simulink model "model6krata"  (Simulink 6.6)
settings: Solver=ode45  StartTime=0.0  StopTime=700  MaxStep=0.01  MinStep=0.001  RelTol=1e-6
values from neighbouring files (symbols this model uses):
  c1 = 8    [dane6krata.m]
  c2 = 5    [dane6krata.m]
  mi1 = 1    [dane6krata.m]
  mi2 = 2    [dane6krata.m]
  q = 1    [dane6krata.m]
undefined symbols (not defined in the file or in its folder): sgn
settings Model: Creator=Administrator  LastModifiedBy=Damian
settings DataIOCC: LimitDataPoints=off
settings GRTTargetCC: TargetFcnLib=ansi_tfl_table_tmw.mat

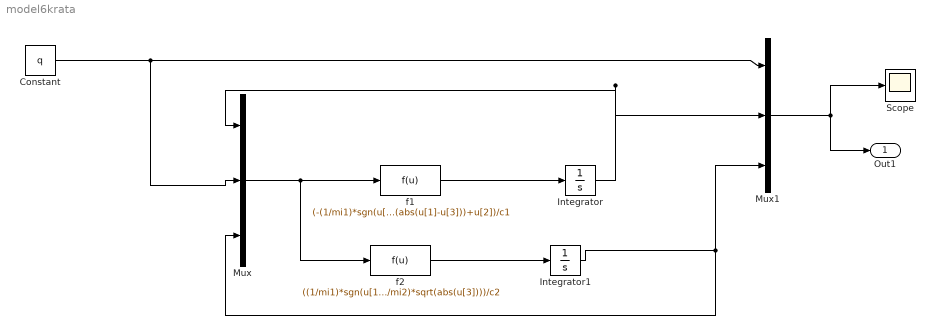
== system model6krata ==
  Constant : Constant  Value=q
  Integrator : Integrator
  Integrator1 : Integrator
  Mux : Mux  Inputs=3
  Mux1 : Mux  Inputs=3
  Scope : Scope
  f1 : Fcn  Tag=f1  Expr=(-(1/mi1)*sgn(u[1]-u[3])*sqrt(abs(u[1]-u[3]))+u[2])/c1
  f2 : Fcn  Expr=((1/mi1)*sgn(u[1]-u[3])*sqrt(abs(u[1]-u[3]))-(1/mi2)*sqrt(abs(u[3])))/c2
  Out1 : Outport
  wires:
  Mux/1 -> f1/1, f2/1
  f2/1 -> Integrator1/1
  f1/1 -> Integrator/1
  Constant/1 -> Mux1/1, Mux/2
  Integrator/1 -> Mux/1, Mux1/2
  Integrator1/1 -> Mux/3, Mux1/3
  Mux1/1 -> Scope/1, Out1/1
